simulink model "tilp_fxp"  (R2013b)
settings: Solver=FixedStepDiscrete  StartTime=0.0  StopTime=1  FixedStep=0.01  RelTol=1e-3
PreLoadFcn:
  | cordic = 1;
libraries: simulink x1
settings Model: Creator=bas  LastModifiedBy=peselnikmg
settings DataIOCC: SaveOutput=off  DSMLogging=off  InspectSignalLogs=on  SaveTime=off
settings OptimizationCC: ExpressionDepthLimit=2147483647  OptimizeModelRefInitCode=on  LifeSpan=Inf
settings DebuggingCC: FcnCallInpInsideContextMsg=EnableAllAsWarning  StateNameClashWarn=warning
settings HardwareCC: ProdBitPerInt=16  ProdBitPerPointer=16  ProdIntDivRoundTo=Zero  ProdEndianess=LittleEndian  ProdWordSize=16  ProdHWDeviceType=Texas Instruments->MSP430
settings RTWCC: SystemTargetFile=launchpad.tlc  TemplateMakefile=launchpad_tmf  Description=TI LaunchPad  GenerateReport=on  ProcessScript=launchpad_make_rtw_hook  IncludeHyperlinkInReport=on  PortableWordSizes=on  CodeExecutionProfiling=on  CodeProfilingSaveOptions=AllData  GenerateTraceInfo=on  GenerateTraceReport=on  GenerateTraceReportSl=on  GenerateTraceReportSf=on  GenerateTraceReportEml=on
settings CodeAppCC: IgnoreCustomStorageClasses=off  CustomSymbolStrType=$N$R$M  InternalIdentifier=Classic
settings STFCustomTargetCC: CombineOutputUpdateFcns=on  ERTCustomFileBanners=on  SupportContinuousTime=off  SupportNonInlinedSFcns=off  MATLABClassNameForMDSCustomization=Simulink.SoftwareTarget.ERTCustomization  GRTInterface=off  SystemTargetFile=launchpad.tlc
settings ERTTargetCC: CodeReplacementLibrary=ANSI_C  ParMdlRefBuildCompliant=off  CompOptLevelCompliant=off  ConcurrentExecutionCompliant=off  ERTFirstTimeCompliant=off  ModelStepFunctionPrototypeControlCompliant=off  CPPClassGenCompliant=off  ExtModeMexFile=noextcomm  InlinedParameterPlacement=NonHierarchical  ERTCustomFileTemplate=launchpad_srmain.tlc

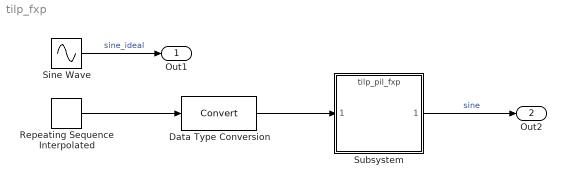
== system tilp_fxp ==
  Data Type Conversion : DataTypeConversion
  Repeating Sequence Interpolated : simulink/Sources/Repeating Sequence Interpolated  OutValues=linspace(-2*pi,2*pi,100)'  TimeValues=linspace(0,1,100)'  LookUpMeth=Interpolation-Use End Values  tsamp=0.01  OutMin=[]  OutMax=[]  OutDataTypeStr=double  OutputDataTypeScalingMode=double  OutDataType=fixdt(0,8)  OutScaling=2^-10
  Sine Wave : Sin  Frequency=4*pi  SampleTime=0
  Subsystem : ModelReference  ModelNameDialog=tilp_pil_fxp  SimulationMode=Processor-in-the-loop (PIL)  ModelReferenceVersion=1.451  CopyOfModelName=tilp_pil_fxp  DefaultDataLogging=on
  Out1 : Outport
  Out2 : Outport  Port=2
  wires:
  Subsystem/1 -> Out2/1  "sine"
  Repeating Sequence Interpolated/1 -> Data Type Conversion/1
  Data Type Conversion/1 -> Subsystem/1
  Sine Wave/1 -> Out1/1  "sine_ideal"
